simulink model "eg"  (R2018b)
settings: Solver=VariableStepAuto  StartTime=0.0  StopTime=10  RelTol=1e-3
libraries: dsparch4 x2, commrandsrc3 x1
settings Model: Creator=lance  LastModifiedBy=lance

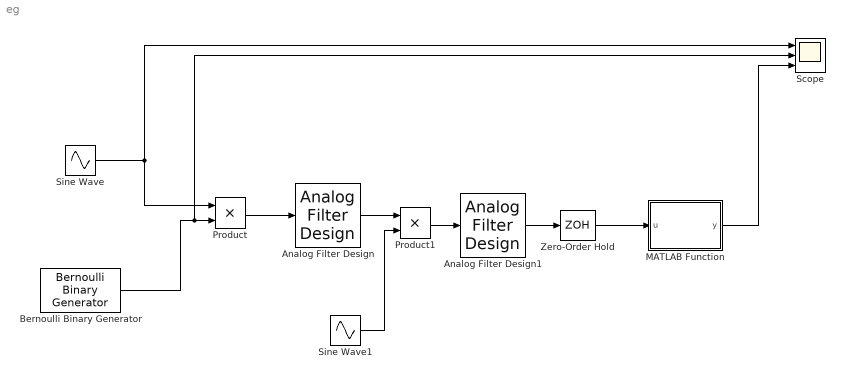
== system eg ==
  Analog Filter Design : dsparch4/Analog Filter Design  method=Butterworth  filttype=Bandpass  N=8  Wlo=97*2*pi  Whi=103*2*pi  Rp=2  Rs=40
  Analog Filter Design1 : dsparch4/Analog Filter Design  method=Butterworth  filttype=Lowpass  N=8  Wlo=2*pi  Whi=103*2*pi  Rp=2  Rs=40
  Bernoulli Binary Generator : commrandsrc3/Bernoulli Binary Generator  ProbabilityOfZero=0.5  SeedSource=Parameter  Seed=61  SampleTime=1  SamplesPerFrame=1  OutputDataType=double  SimulateUsing=Interpreted execution
  MATLAB Function : MATLAB Function  TreatAsAtomicUnit=on
  Product : Product
  Product1 : Product
  Scope : Scope  NumInputPorts=3
  Sine Wave : Sin  Frequency=100*2*pi  SampleTime=0.0001
  Sine Wave1 : Sin  Frequency=100*2*pi  SampleTime=0.0001
  Zero-Order Hold : ZeroOrderHold
  wires:
  Sine Wave/1 -> Scope/1, Product/1
  Bernoulli Binary Generator/1 -> Scope/2, Product/2
  Product/1 -> Analog Filter Design/1
  Sine Wave1/1 -> Product1/2
  Analog Filter Design/1 -> Product1/1
  Product1/1 -> Analog Filter Design1/1
  Analog Filter Design1/1 -> Zero-Order Hold/1
  Zero-Order Hold/1 -> MATLAB Function/1(u)
  MATLAB Function/1(y) -> Scope/3

== matlab function eg/MATLAB Function ==
  data: u input; y output
function y = fcn(u)
if(u>0.24)
    y=1;
else
    y=0;
end
